simulink model "MMMS_v3"  (R2024b)
settings: Solver=VariableStepAuto  StartTime=0.0  StopTime=60  FixedStep=0.001  RelTol=1e-3
InitFcn:
  | %rho_0t=[0.29;0.29;0.29]; %m
  | %V_0t=[-0.001;-0.001;0];%[-0.0005;-0.0005;0];
  | %w_t=[0;0;-0.002];
  | 
  | 
  | %rho_0t=[0.3;0.3;0.2]; %m
  | %V_0t=[-0.001;-0.001;0];%[-0.0005;-0.0005;0];
  | %w_t=[0;0;-0.001];
values from neighbouring files (symbols this model uses):
  Dt = 0.1    [main_EKF.m]
  Fake_Manip_grad = -0.2.*eye(7)    [Initiate_FQ.m]
  g_cm = zeros(4,4,n)    [Initiate_KUKA_inv.m]    (also in Main_MMMS.m; test_KUKA_elements.m)
  g_It00 = [eye(3) rho_It;0 0 0 1]    [main_EKF.m]
  iota0 = eye(6,6)    [Initiate_KUKA_inv.m]    (also in Main_MMMS.m; test_KUKA_elements.m)
  K_d = 10*[1.3*eye(3) zeros(3);zeros(3) 0.8*eye(3)]    [Initiate_FQ.m]    (also in Initiate_KUKA_inv.m = 5*[0.7*eye(3) zeros(3);zeros(3) 0.5*eye(3)]; MMMS_Initiate_FQ.m; Main_MMMS.m = 5*[0.7*eye(3) zeros(3);zeros(3) 0.5*eye(3)]; test_KUKA_elements.m = 50*[0.7*eye(3) zeros(3);zeros(3) 0.5*eye(3)])
  K_i = 5*[0.1*eye(3) zeros(3);zeros(3) 0.01*eye(3)]    [Initiate_FQ.m]    (also in Initiate_KUKA_inv.m = 5*[0.01*eye(3) zeros(3);zeros(3) 0.001*eye(3)]; MMMS_Initiate_FQ.m; Main_MMMS.m = 5*[0.01*eye(3) zeros(3);zeros(3) 0.001*eye(3)]; test_KUKA_elements.m = 50*[0.01*eye(3) zeros(3);zeros(3) 0.001*eye(3)])
  K_p = 100*[0.1 0 0 0 0 0;0 0.1 0 0 0 0; 0 0 0.1 0 0 0; 0 0 0 0.01 0 0 ... (first row only)    [Initiate_FQ.m]    (also in Initiate_KUKA_inv.m = 5*[0.1 0 0 0 0 0;0 0.1 0 0 0 0; 0 0 0.1 0 0 0; 0 0 0 0.01 0 ; MMMS_Initiate_FQ.m; Main_MMMS.m = 5*[0.1 0 0 0 0 0;0 0.1 0 0 0 0; 0 0 0.1 0 0 0; 0 0 0 0.01 0 ; test_KUKA_elements.m = 50*[0.1 0 0 0 0 0;0 0.1 0 0 0 0; 0 0 0.1 0 0 0; 0 0 0 0.01 0)
  K_w = 200*eye(7)    [Initiate_FQ.m]    (also in MMMS_Initiate_FQ.m)
  K_wd = 2*eye(7)    [Initiate_FQ.m]    (also in MMMS_Initiate_FQ.m)
  m = randn(s,total_time_steps,6)*chol(R)    [main_EKF.m]
  M0 = M_temp.M0.data(:,:,1)    [Initiate_FQ.m]    (also in MMMS_Initiate_FQ.m; test_KUKA_elements.m)
  m0 = robot.Bodies{1,n+1}.Mass    [Initiate_KUKA_inv.m]    (also in Main_MMMS.m; test_KUKA_elements.m)
  m0_frak = diag_M(1:6,1:6)    [Initiate_KUKA_inv.m]    (also in Main_MMMS.m; make_uncertain.m = diag_M_unc(1:6,1:6); test_KUKA_elements.m)
  M0m = M_temp.M0m.data(:,:,1)    [Initiate_FQ.m]    (also in MMMS_Initiate_FQ.m; test_KUKA_elements.m)
  m_diag = diag_M(7:end,7:end)    [Initiate_KUKA_inv.m]    (also in Main_MMMS.m; make_uncertain.m = diag_M_unc(7:end,7:end); test_KUKA_elements.m)
  M_t = (((Adjoint(g_It))'\M_t_body)/(Adjoint(g_It)))    [Initiate_FQ.m]    (also in Initiate_KUKA_inv.m = [eye(3)*mt zeros(3); zeros(3) eye(3)*80]; MMMS_Initiate_FQ.m; Main_MMMS.m = [eye(3)*mt zeros(3); zeros(3) eye(3)*80]; test_KUKA_elements.m = [eye(3)*mt zeros(3); zeros(3) eye(3)*80])
  M_t_body = [eye(3)*mt zeros(3); zeros(3) eye(3)*0.416667]    [Initiate_FQ.m]    (also in MMMS_Initiate_FQ.m)
  mm = zeros(1,n)    [Initiate_KUKA_inv.m]    (also in Main_MMMS.m; test_KUKA_elements.m)
  mu = P0    [Initiate_FQ.m]    (also in Initiate_KUKA_inv.m = zeros(6,1); MMMS_Initiate_FQ.m; Main_MMMS.m = zeros(6,1); make_uncertain.m = P0_unc)
  mu_t = inv((Adjoint(g_It))')*M_t_body*[V_It;w_t]    [Initiate_FQ.m]    (also in Initiate_KUKA_inv.m = M_t*[V_0t;w_t]; MMMS_Initiate_FQ.m; Main_MMMS.m = M_t*[V_0t;w_t]; make_uncertain.m = inv((Adjoint(g_It))')*M_t_body_unc*[V_It;w_t])
  noise_st = 0.000005    (= 5e-06)    [main_EKF.m]
  q_dot_m = [0;0;0;0;0;0;0]    [Initiate_FQ.m]    (also in Initiate_KUKA_inv.m; MMMS_Initiate_FQ.m; Main_MMMS.m; test_KUKA_elements.m = [0])
  q_m = [0.2;1.2;0.3;2.5;0.5;1.5;0.6]    [Initiate_FQ.m]    (also in Initiate_KUKA_inv.m = [0;0;0;0;0;0;0]; MMMS_Initiate_FQ.m = [0.2;0.2;0.3;0.5;0.5;0.5;0.6]; Main_MMMS.m = [0;0;0;0;0;0;0]; test_KUKA_elements.m = [0.2;1.2;0.3;1.8;0.5;1.3;0.6])
  rho_It = [0;0;1.7]    [Initiate_FQ.m]    (also in MMMS_Initiate_FQ.m)
  s = RandStream.create('mrg32k3a','NumStreams',1)    [main_EKF.m]
  sc_size = 1    [Initiate_KUKA_inv.m]    (also in Main_MMMS.m; test_KUKA_elements.m)
  V_It = [0.0005;0.0005;0]    [Initiate_FQ.m]    (also in MMMS_Initiate_FQ.m = [0.001;0.001;0])
  Xi_m_matrix = zeros(6*n,n)    [Initiate_KUKA_inv.m]    (also in Main_MMMS.m)
undefined symbols (not defined in the file or in its folder): g_cm0, I0, Im, Mm, X, Xi_m, Y, Z
libraries: nesl_utility x314, sm_lib x231, robotcorelib x30, simulink x12
(part 13 of 13)

== matlab function MMMS_v3/Feedback Transformation2/Inverse Dynamics1/C_hat1/M_partials1/M0mpartial ==
  data: q_m input; M0m_partial output; V input; Lm input; Lm0 input; iota0 input; diag_Mm input; Lm0_partial input; Lm_partial input; Xi_m_matrix input
function M0m_partial = M0m_partial(q_m,V,Lm,Lm0,iota0,diag_Mm,Lm0_partial,Lm_partial, Xi_m_matrix)
% Calculates the C_hat_m matrix from base pose and arm joint angles

n=length(q_m);
b=length(V);

% Find partial of M0m to joint angles
M0m_partial=zeros(b,n,n);
for i=1:n
    temp1=transpose(Lm0_partial(1:end,1:end,i))*diag_Mm*Lm;
    temp2=transpose(Lm0)*diag_Mm*Lm_partial(1:end,1:end,i);
    M0m_partial(1:b,1:n,i)= iota0'*(temp1+temp2)*Xi_m_matrix; % equation 118 of TRO paper
end

== matlab function MMMS_v3/Feedback Transformation2/Inverse Dynamics1/C_hat1/M_partials1/M0mpartial_par ==
  data: q_m input; M0m_partial_par output; V input; Lm input; Lm0 input; iota0 input; diag_Mm input; Lm0_partial input; Lm_partial input; Xi_m_matrix input; Lm0_partial_par input; Lm_partial_par input
function M0m_partial_par = M0m_partial_par(q_m,V,Lm,Lm0,iota0,diag_Mm,Lm0_partial,Lm_partial, Xi_m_matrix,Lm0_partial_par,Lm_partial_par)
% Calculates the C_hat_m matrix from base pose and arm joint angles

n=length(q_m);
b=length(V);

% Find partial of M0m to joint angles
M0m_partial_par=zeros(b,n,n,n);
for i=1:n
    for s=1:n
        temp1=transpose(Lm0_partial_par(1:end,1:end,i,s))*diag_Mm*Lm;
        temp2=transpose(Lm0_partial(1:end,1:end,i))*diag_Mm*Lm_partial(1:end,1:end,s);
        temp3=transpose(Lm0_partial(1:end,1:end,s))*diag_Mm*Lm_partial(1:end,1:end,i);
        temp4=transpose(Lm0)*diag_Mm*Lm_partial_par(1:end,1:end,i,s);
        M0m_partial_par(1:b,1:n,i,s)= iota0'*(temp1+temp2+temp3+temp4)*Xi_m_matrix; % equation 118 of TRO paper
    end
end


% M0m_partial_par

== matlab function MMMS_v3/Feedback Transformation2/Inverse Dynamics1/C_hat1/M_partials1/Mmpartial ==
  data: q_m input; Mm_partial output; Xi_m_matrix input; Lm input; diag_Mm input; Lm_partial input
function Mm_partial = Mm_partial(q_m,Xi_m_matrix,Lm,diag_Mm,Lm_partial)
% Calculates the C_hat_m matrix from base pose and arm joint angles

n=length(q_m);

% find the non-generalized arm mass matrix'x derivative to joint angles
Mm_partial=zeros(n,n,n);
for i=1:n
    temp=   transpose(Lm_partial(1:6*n,1:6*n,i))*diag_Mm*Lm  +   transpose(Lm)*diag_Mm*Lm_partial(1:6*n,1:6*n,i);
    Mm_partial(1:n,1:n,i)=transpose(Xi_m_matrix)*temp*Xi_m_matrix; %calcualte the derivative of not-augmented arm mass matrix from equation 120 of TRO paper
end

== matlab function MMMS_v3/Feedback Transformation2/Inverse Dynamics1/C_hat1/Mm_hat_partial1 ==
  data: q_m input; AMA_partial input; Mm_hat_partial output; Mm_partial input
function Mm_hat_partial = Mm_hat_partial(q_m, AMA_partial, Mm_partial)
% Calculates the C_hat_m matrix from base pose and arm joint angles

n=length(q_m);

% find the generalized arm mass matrix'x derivative to joint angles
Mm_hat_partial=zeros(n,n,n);
for i=1:n
    Mm_hat_partial(1:n,1:n,i)=Mm_partial(1:n,1:n,i)-AMA_partial(1:n,1:n,i); %calcualte the derivative of augmented arm mass matrix from equation 119 of TRO paper
end

== matlab function MMMS_v3/Controller23/sensing noise in g_t ==
  data: err input; errM output
function errM = fcn(err)

errM=expm(wedge(err));

== matlab function MMMS_v3/Inverse Dynamics/N_hat1/MATLAB Function ==
  data: g_I0 input; V_Ie output; V_Ie_e input
function V_Ie = fcn(g_I0,V_Ie_e)

V_Ie = Adjoint(g_I0)\V_Ie_e;

== matlab function MMMS_v3/Controller23/V_It_2 ==
  data: mu_t input; M_t_body input; g_It input; V_It_2 output
function V_It_2 = V_It(mu_t, M_t_body, g_It)


% g_gpt=[eye(3) [0.25; 0.25; 0.25]; 0 0 0 1];
R=g_It(1:3,1:3);

% Pt=(Adjoint(g_It))'*mu_t;
V_It_2=(Adjoint(g_It))*inv(M_t_body)*(Adjoint(g_It)')*mu_t;%Adjoint(g_It)*M_t_body\Pt;%(Mt\(Adjoint(g_It)')*Pt); %[R zeros(3);zeros(3) R]



% Ad g_Igp(t) M^-1 Ad gI_gp(t)' inv(Ad g_I_gp') Mt inv (Ad g_I_gp) V_Igp

== matlab function MMMS_v3/Inverse Dynamics/C_hat1/AMA_partial ==
  data: q_m input; AMA_partial output; M0 input; A input; A_partial input; V input; M0_partial input
function AMA_partial = AMA_partial(q_m,M0,A,A_partial,V,M0_partial)
% Calculates the C_hat_m matrix from base pose and arm joint angles

n=length(q_m);
b=length(V);

% find the temp intermediate term
AMA_partial=zeros(n,n,n);
for i=1:n
    AMA_partial(1:n,1:n,i)=transpose(A_partial(1:end,1:end,i))*M0*A+transpose(A)*M0_partial(1:end,1:end,i)*A+transpose(A)*M0*A_partial(1:end,1:end,i); %calcualte the derivative of not-augmented arm mass matrix from equation 121 of TRO paper
end

== matlab function MMMS_v3/Inverse Dynamics/C_hat1/A_partial ==
  data: q_m input; A_partial output; M0 input; M0_partial input; M0m_partial input; M0m input; V input
function A_partial = A_partial(q_m,M0,M0_partial,M0m_partial,M0m,V)
% Calculates the C_hat_m matrix from base pose and arm joint angles

n=length(q_m);
b=length(V);

% Find partial of connection A to each joint angle
A_partial=zeros(b,n,n);

temp1=zeros(b,n);
temp2=zeros(b,n);
temp3=zeros(b,n);

for i=1:n
    temp1=M0\M0_partial(1:end,1:end,i);
    temp2=M0\M0m;
    temp3=M0\M0m_partial(1:end,1:end,i);
    A_partial(1:b,1:n,i)=-temp1*temp2+temp3; % Equation 122
end

== matlab function MMMS_v3/Controller23/Potential Function ==
  data: U_ff output; A input; w input; grad_w input; U_c input; p_0n input; sc_size input; Mm_hat input; g_n0 input
function U_ff = U_ff(A,w,grad_w, U_c, p_0n, sc_size,Mm_hat, g_n0)


grad_w_p=p_0n/(norm(p_0n)); % d/dt(1/sqrt(x^2+y^2+z^2)) = -1/2*w_p^3 * d/dt (x^2+...)
w_lim=0.003;
w_p_lim=0.02;
r_lim=sqrt(2)*sc_size/2+0.02;

w_p=norm(p_0n)-r_lim;

JJ=A;
A_dagger = ((Mm_hat)\JJ')/((JJ/Mm_hat)*JJ');

if w<w_lim %--------------------------------------------- close to singular
%     temp=(pinv(A)'*grad_w);
%     dir=(temp)./(norm(temp));
%     Uc=U_c-dot(U_c,dir).*dir;

    if w_p<w_p_lim %-------------- EE collision w Spacecraft
        if w_p<w_p_lim/4
            U_c=U_c-dot(U_c,[(grad_w_p); zeros(3,1)]);
        end
        U_c=U_c-10.*(1-w_p_lim/w_p)*((w_p_lim)/w_p^2).*[(grad_w_p); zeros(3,1)]; %(1/(1+100*exp(1000*(w_p-(sqrt(2)*sc_size/2+0.05)))))*2*
    end
    
    U_ff=U_c-((1-w_lim/w)*(w_lim/w^2).*A_dagger'*grad_w); %1*(1-w_lim/w)*
    %(1/(1+100*exp(1000*(w-0.003))))*0.0001*pinv(A)'*(-grad_w./(w^2)); 
    %adjoint_low(Adjoint(g_I0)*V_Ie)*Adjoint(inv(g_I0))*V_It+Adjoint(inv(g_I0))*V_It_dot

else %----------------------------------------------- NOT close to singular
    
    if w_p<w_p_lim %-------------- EE collision w Spacecraft
        if w_p<w_p_lim/4
            U_c=U_c-dot(U_c,[(grad_w_p); zeros(3,1)]);
        end
        U_c=U_c-10.*(1-w_p_lim/w_p)*((w_p_lim)/w_p^2).*[(grad_w_p); zeros(3,1)];
        %(1/(1+100*exp(1000*(w_p-(sqrt(2)*sc_size/2+0.05)))))*2*
        
    end

    U_ff=U_c;
end

== matlab function MMMS_v3/Controller23/mu_init ==
  data: g_It input; Mt input; V_It input; mu_init output
function mu_init = mu_init(g_It,Mt,V_It)

mu_init=Mt*V_It; %*(inv(Adjoint(g_It)))


% Ad g_Igp(t) M^-1 Ad gI_gp(t)' inv(Ad g_I_gp') Mt inv (Ad g_I_gp) V_Igp

== matlab function MMMS_v3/Controller23/V_It_1 ==
  data: V_It input; g_It input; V_It_3 output
function V_It_3 = V_It3(V_It, g_It)


% g_gpt=[eye(3) [0.25; 0.25; 0.25]; 0 0 0 1];
R=g_It(1:3,1:3);

V_It_3=Adjoint(g_It)*[R zeros(3);zeros(3) R]'*V_It; %[R zeros(3);zeros(3) R]


% Ad g_Igp(t) M^-1 Ad gI_gp(t)' inv(Ad g_I_gp') Mt inv (Ad g_I_gp) V_Igp

== matlab function MMMS_v3/Controller23/Kinematics/MATLAB Function ==
  data: g_I0 input; V_Ie output; V_Ie_e input
function V_Ie = fcn(g_I0,V_Ie_e)

V_Ie = Adjoint(g_I0)*V_Ie_e;

== matlab function MMMS_v3/Controller23/Filter/sensing noise in g_t1 ==
  data: z input; errM output; z_gt input
function errM = fcn(z,z_gt)

g_te=(z\z_gt);

R_te=g_te(1:3,1:3);
p_te=g_te(1:3,4);

temp_R=eye(3)-R_te;
temp_R=0.5*trace(temp_R);

temp_p=0.5*transpose(p_te)*p_te;
errM =temp_R+temp_p;

== matlab function MMMS_v3/Dynamic Parameters/ 1 ==
  data: q_m input; L0 output; Lm0 output; Lm output; Xi_m input
function [L0,Lm0,Lm] =L_calculator(q_m,Xi_m)
% Calculates the time-dependent L matrix
n=length(q_m);
L=zeros(6*(n+1),6*(n+1));
% Compute M_frak for ith body
% Calculate L matrix
for i=1:n+1
    for j=1:n+1
        if i>j
            Ad_temp=eye(6);
            for k=j:i-1
                Ad_temp=Adjoint(g_Matrix(-Xi_m(:,k),q_m(k)))*Ad_temp;
            end
            L(6*(i-1)+1:6*(i-1)+6,6*(j-1)+1:6*(j-1)+6)=Ad_temp;
        elseif i==j
            L(6*(i-1)+1:6*(i-1)+6,6*(j-1)+1:6*(j-1)+6)=eye(6);
        elseif i<j
            L(6*(i-1)+1:6*(i-1)+6,6*(j-1)+1:6*(j-1)+6)=zeros(6);
        end
    end
end

L0=L(1:6,1:6);
Lm0=L(7:end,1:6);
Lm=L(7:end,7:end);

end

== matlab function MMMS_v3/Controller23/Filter/sensing noise in g_t2 ==
  data: z input; errM output; z_gt input
function errM = fcn(z,z_gt)

g_te=(z\z_gt);

R_te=g_te(1:3,1:3);
p_te=g_te(1:3,4);

temp_R=eye(3)-R_te;
temp_R=0.5*trace(temp_R);

temp_p=0.5*transpose(p_te)*p_te;
errM =temp_R+temp_p;

== matlab function MMMS_v3/Inverse Dynamics/C_hat1/C_hat ==
  data: q_m input; Mm_hat_partial input; q_dot_m input; C_hat output
function C_hat = C_hat(q_m, Mm_hat_partial,q_dot_m)
% Calculates the C_hat_m matrix from base pose and arm joint angles

n=length(q_m);


% Calculate C_hat matrix
C_temp1=zeros(n,n);
C_temp2=zeros(n,n);
C_hat=zeros(n,n);
for i=1:n
    C_temp1=C_temp1+squeeze(Mm_hat_partial(1:n,1:n,i)).*q_dot_m(i); % nxn by scalar
    C_temp2(i,1:n)=0.5*transpose(q_dot_m)*squeeze(Mm_hat_partial(1:n,1:n,i)); %1xn by nxn 
end

C_hat=C_temp1-C_temp2;

== matlab function MMMS_v3/Controller23/  ==
  data: A input; normA output
function normA  = normA(A)

normA=norm(A);

== matlab function MMMS_v3/MMS3/collect positions ==
  data: p_ni output; p_n2 input; p_n3 input; p_n4 input; p_n5 input; g_n0 input
function p_ni = collect_positions(p_n2,p_n3,p_n4,p_n5, g_n0)

% R_0n=g_n0(1:3,1:3);
% p_0n=g_n0(1:3,4);

% p_joints=zeros(3,5);
p_ni=[p_n2 p_n3 p_n4  p_n5];
% p_joints=p_joints_temp(1:3,:);

== matlab function MMMS_v3/MMS3/collect positions1 ==
  data: g_ni output; g_n2 input; g_n3 input; g_n4 input; g_n5 input; g_n0 input
function g_ni = collect_poses(g_n2,g_n3,g_n4,g_n5, g_n0)

g_ni=zeros(4,4,4);
% p_joints=zeros(3,5);
g_ni(1,:,:)=g_n2;
g_ni(2,:,:)=g_n3;
g_ni(3,:,:)=g_n4;
g_ni(4,:,:)=g_n5;

== matlab function MMMS_v3/MMS4/collect positions ==
  data: p_ni output; p_n2 input; p_n3 input; p_n4 input; p_n5 input; g_n0 input
function p_ni = collect_positions(p_n2,p_n3,p_n4,p_n5, g_n0)

% R_0n=g_n0(1:3,1:3);
% p_0n=g_n0(1:3,4);

% p_joints=zeros(3,5);
p_ni=[p_n2 p_n3 p_n4  p_n5];
% p_joints=p_joints_temp(1:3,:);

== matlab function MMMS_v3/Inverse Dynamics/C_hat1/Lm_partials/Lm0partial ==
  data: q_m input; Lm0_partial output; Xi_m input; iota0 input
function Lm0_partial = Lm0_partial(q_m,Xi_m,iota0)
% Calculates the C_hat_m matrix from base pose and arm joint angles

n=length(q_m);

% Find partial of Lm to joint angles
Lm0_partial=zeros(6*n,6,n); % 6nx6xn
for i=1:n
    for j=1:n
        Lm0_partial(6*(j-1)+1:6*j,1:6,i)=Ad_partial(j,1,i,Xi_m,q_m,iota0); % equation 114 of TRO paper
    end
end

%%%%%%%%%%%%%%%%%%%%%%%%%%%%%%%%%%%%%%%%%%%%%%%%%%%%%%%%%%%%% MUST BE
%%%%%%%%%%%%%%%%%%%%%%%%%%%%%%%%%%%%%%%%%%%%%%%%%%%%%%%%%%%%% CHECKED

== matlab function MMMS_v3/MMS4/collect positions1 ==
  data: g_ni output; g_n2 input; g_n3 input; g_n4 input; g_n5 input; g_n0 input
function g_ni = collect_poses(g_n2,g_n3,g_n4,g_n5, g_n0)

g_ni=zeros(4,4,4);
% p_joints=zeros(3,5);
g_ni(1,:,:)=g_n2;
g_ni(2,:,:)=g_n3;
g_ni(3,:,:)=g_n4;
g_ni(4,:,:)=g_n5;

== matlab function MMMS_v3/Controller1/  ==
  data: A input; normA output
function normA  = normA(A)

normA=norm(A);

== matlab function MMMS_v3/Dynamic Parameters1/ 1 ==
  data: q_m input; L0 output; Lm0 output; Lm output; Xi_m input
function [L0,Lm0,Lm] =L_calculator(q_m,Xi_m)
% Calculates the time-dependent L matrix
n=length(q_m);
L=zeros(6*(n+1),6*(n+1));
% Compute M_frak for ith body
% Calculate L matrix
for i=1:n+1
    for j=1:n+1
        if i>j
            Ad_temp=eye(6);
            for k=j:i-1
                Ad_temp=Adjoint(g_Matrix(-Xi_m(:,k),q_m(k)))*Ad_temp;
            end
            L(6*(i-1)+1:6*(i-1)+6,6*(j-1)+1:6*(j-1)+6)=Ad_temp;
        elseif i==j
            L(6*(i-1)+1:6*(i-1)+6,6*(j-1)+1:6*(j-1)+6)=eye(6);
        elseif i<j
            L(6*(i-1)+1:6*(i-1)+6,6*(j-1)+1:6*(j-1)+6)=zeros(6);
        end
    end
end

L0=L(1:6,1:6);
Lm0=L(7:end,1:6);
Lm=L(7:end,7:end);

end

== matlab function MMMS_v3/Dynamic Parameters1/MATLAB Function ==
  data: A input; wt output
function wt = fcn(A)

J=-A;
% SVD=svd(J);

% minSVD=min(SVD);
% maxSVD=max(SVD);

wt=sqrt(det(J*J'));

% y = minSVD/maxSVD;

== matlab function MMMS_v3/Controller23/gradient_of_Eg ==
  data: g_te input; Nabla_Eg output
function Nabla_Eg = fcn(g_te)

% Calculate the gradient of the Pose Error Function
p_te=g_te(1:3,4);
R_te=g_te(1:3,1:3);

temp=0.5*(R_te-transpose(R_te));

R_temp=vee3(temp);

Nabla_Eg=[p_te;R_temp];

== matlab function MMMS_v3/Inverse Dynamics/C_hat1/Lm_partials/Lmpartial ==
  data: q_m input; Lm_partial output; Xi_m input; iota0 input
function Lm_partial  = Lm_partial(q_m,Xi_m,iota0)
% Calculates the C_hat_m matrix from base pose and arm joint angles

n=length(q_m);

% Find partial of Lm0 to joint angles
Lm_partial=zeros(6*n,6*n,n); % 6nx6xn
for i=1:n
    Lm_partial(:,:,i)=zeros(6*n,6*n);
    for j=2:n
        for k=2:n
            if j>i && i>=k
                Lm_partial(6*(j-1)+1:6*j,6*(k-2)+1:6*(k-1),i)=Ad_partial(j,k,i,Xi_m,q_m,iota0); % equation 81 of TRO paper
            elseif i==j && i>=k
                Lm_partial(6*(j-1)+1:6*j,6*(k-2)+1:6*(k-1),i)=Ad_partial(j,k,i,Xi_m,q_m,iota0); % equation 81 of TRO paper
            else
                Lm_partial(6*(j-1)+1:6*(j-1)+6,6*(k-2)+1:6*(k-2)+6,i)=zeros(6,6);
            end

        end
    end
end

== matlab function MMMS_v3/Inverse Dynamics/C_hat1/M_partials/ M0partial ==
  data: q_m input; M0_partial output; Lm0 input; V input; iota0 input; diag_Mm input; Lm0_partial input
function M0_partial = M0_partial(q_m,Lm0,V,iota0,diag_Mm,Lm0_partial)
% Calculates the C_hat_m matrix from base pose and arm joint angles

n=length(q_m);
b=length(V);

% Find partial of M0 to joint angles
M0_partial=zeros(b,b,n); %initiate
for i=1:n
    temp1=transpose(Lm0_partial(1:end,1:end,i))*diag_Mm*Lm0;
    temp2=transpose(Lm0)*diag_Mm*Lm0_partial(1:end,1:end,i);
    M0_partial(1:b,1:b,i)= iota0'*(temp1+temp2)*iota0; %6x6 %equation 117 of TRO
end

== matlab function MMMS_v3/Inverse Dynamics/C_hat1/M_partials/M0mpartial ==
  data: q_m input; M0m_partial output; V input; Lm input; Lm0 input; iota0 input; diag_Mm input; Lm0_partial input; Lm_partial input; Xi_m_matrix input
function M0m_partial = M0m_partial(q_m,V,Lm,Lm0,iota0,diag_Mm,Lm0_partial,Lm_partial, Xi_m_matrix)
% Calculates the C_hat_m matrix from base pose and arm joint angles

n=length(q_m);
b=length(V);

% Find partial of M0m to joint angles
M0m_partial=zeros(b,n,n);
for i=1:n
    temp1=transpose(Lm0_partial(1:end,1:end,i))*diag_Mm*Lm;
    temp2=transpose(Lm0)*diag_Mm*Lm_partial(1:end,1:end,i);
    M0m_partial(1:b,1:n,i)= iota0'*(temp1+temp2)*Xi_m_matrix; % equation 118 of TRO paper
end

== matlab function MMMS_v3/Inverse Dynamics/C_hat1/M_partials/Mmpartial ==
  data: q_m input; Mm_partial output; Xi_m_matrix input; Lm input; diag_Mm input; Lm_partial input
function Mm_partial = Mm_partial(q_m,Xi_m_matrix,Lm,diag_Mm,Lm_partial)
% Calculates the C_hat_m matrix from base pose and arm joint angles

n=length(q_m);

% find the non-generalized arm mass matrix'x derivative to joint angles
Mm_partial=zeros(n,n,n);
for i=1:n
    temp=   transpose(Lm_partial(1:6*n,1:6*n,i))*diag_Mm*Lm  +   transpose(Lm)*diag_Mm*Lm_partial(1:6*n,1:6*n,i);
    Mm_partial(1:n,1:n,i)=transpose(Xi_m_matrix)*temp*Xi_m_matrix; %calcualte the derivative of not-augmented arm mass matrix from equation 120 of TRO paper
end

== matlab function MMMS_v3/Inverse Dynamics/C_hat1/Mm_hat_partial ==
  data: q_m input; AMA_partial input; Mm_hat_partial output; Mm_partial input
function Mm_hat_partial = Mm_hat_partial(q_m, AMA_partial, Mm_partial)
% Calculates the C_hat_m matrix from base pose and arm joint angles

n=length(q_m);

% find the generalized arm mass matrix'x derivative to joint angles
Mm_hat_partial=zeros(n,n,n);
for i=1:n
    Mm_hat_partial(1:n,1:n,i)=Mm_partial(1:n,1:n,i)-AMA_partial(1:n,1:n,i); %calcualte the derivative of augmented arm mass matrix from equation 119 of TRO paper
end

== matlab function MMMS_v3/Dynamic Parameters1/MATLAB Function1 ==
  data: g_I0 input; mu input; P output
function P=Momentum(g_I0,mu)
% find the momentum in current base frame
P=Adjoint(g_I0)'*mu;

== matlab function MMMS_v3/Controller23/Kinematics/V_It_1 ==
  data: V_I0 input; g_I0 input; V_I0_3 output
function V_I0_3 = V_I03(V_I0, g_I0)


% g_gpt=[eye(3) [0.25; 0.25; 0.25]; 0 0 0 1];
R=g_I0(1:3,1:3);

V_I0_3=Adjoint(g_I0)*[R zeros(3);zeros(3) R]'*V_I0; %[R zeros(3);zeros(3) R]


% Ad g_Igp(t) M^-1 Ad gI_gp(t)' inv(Ad g_I_gp') Mt inv (Ad g_I_gp) V_Igp

== matlab function MMMS_v3/Controller1/Kinematics/MATLAB Function ==
  data: g_I0 input; V_Ie output; V_Ie_e input
function V_Ie = fcn(g_I0,V_Ie_e)

V_Ie = Adjoint(g_I0)*V_Ie_e;

== matlab function MMMS_v3/Controller13/Kinematics/Pose Error Function ==
  data: g_te input; E_g output
function E_g = pose_Error_function(g_te)
% Calculates the pose Error function from the relative pose of end-effector to target
R_te=g_te(1:3,1:3);
p_te=g_te(1:3,4);

temp_R=eye(3)-R_te;
temp_R=0*0.5*trace(temp_R); %% CHANGED

temp_p=0.5*transpose(p_te)*p_te;
E_g =temp_R+temp_p;

== matlab function MMMS_v3/Controller1/Kinematics/Pose Error Function ==
  data: g_te input; E_g output
function E_g = pose_Error_function(g_te)
% Calculates the pose Error function from the relative pose of end-effector to target
R_te=g_te(1:3,1:3);
p_te=g_te(1:3,4);

temp_R=eye(3)-R_te;
temp_R=0.5*trace(temp_R);

temp_p=0.5*transpose(p_te)*p_te;
E_g =temp_R+temp_p;

== matlab function MMMS_v3/Controller13/Kinematics/Velocity_error ==
  data: g_I0 input; V_Ie input; V_e output; V_It input; g_It input; normV output
function [V_e,normV] = Velocity_Error_function(g_I0, V_Ie,V_It, g_It)
% Calculates the Velocity Error function from the momentums of chaser and
% target and the joint velocities

Rt=g_It(1:3,1:3);
R0=g_I0(1:3,1:3);

V_te_I=V_Ie-V_It; %Adjoint(inv(g_I0))*
V_te=Adjoint(inv(g_I0))*V_te_I;
V_e=V_te;

normV=norm(V_e);

== matlab function MMMS_v3/Controller1/Kinematics/V_It_1 ==
  data: V_I0 input; g_I0 input; V_I0_3 output
function V_I0_3 = V_I03(V_I0, g_I0)


% g_gpt=[eye(3) [0.25; 0.25; 0.25]; 0 0 0 1];
R=g_I0(1:3,1:3);

V_I0_3=Adjoint(g_I0)*[R zeros(3);zeros(3) R]'*V_I0; %[R zeros(3);zeros(3) R]


% Ad g_Igp(t) M^-1 Ad gI_gp(t)' inv(Ad g_I_gp') Mt inv (Ad g_I_gp) V_Igp

== matlab function MMMS_v3/Controller1/Kinematics/Velocity_error ==
  data: g_I0 input; V_Ie input; V_e output; V_It input; g_It input; normV output
function [V_e,normV] = Velocity_Error_function(g_I0, V_Ie,V_It, g_It)
% Calculates the Velocity Error function from the momentums of chaser and
% target and the joint velocities

Rt=g_It(1:3,1:3);
R0=g_I0(1:3,1:3);

V_te_I=V_Ie-V_It; %Adjoint(inv(g_I0))*
V_te=Adjoint(inv(g_I0))*V_te_I;
V_e=V_te;

normV=norm(V_e);

== matlab function MMMS_v3/Controller1/Nullspace derivatives ==
  data: Mm input; A input; N_dot output; Mm_partial input; A_partial input; q_dot input; Z_dot output; j input; Nj input
function [N_dot,Z_dot] =Nullspace_derivatives(Mm,A,Mm_partial,A_partial,q_dot,j, Nj)

Mm_dot=zeros(7);
A_dot=zeros(6,7);
for i=1:length(Mm_partial(1,1,:))
    Mm_dot=Mm_dot+Mm_partial(:,:,i).*q_dot(i);
    A_dot=A_dot+A_partial(:,:,i).*q_dot(i);
end

%parts of N_dot

N1=((Mm\Mm_dot)/Mm)     *   A'   / ((A/Mm)*A')*A;
N2=-Mm\A_dot'   /   ((A/Mm)*A')   * A;
N3=(Mm\A')   /   ((A/Mm)*A')    * ((A_dot/Mm)*A'  -   (A/Mm) *(Mm_dot /Mm) *A'    +   (A/Mm)*A_dot') /   ((A/Mm)*A')   *   A;
N4=-(Mm\ A') *    ((A/Mm)*A')  *A_dot;

N_dot=N1+N2+N3+N4;

% Z_dot=N_dot(:,j);%/norm_Z;
Nj_dot=N_dot(:,j);

Z_dot=Nj_dot/norm(Nj)-Nj'*Nj_dot*Nj/norm(Nj)^3;

== matlab function MMMS_v3/Controller1/Nullspace_maps ==
  data: Mm input; A input; N output; q_dot_m input
function N  =Nullspace_maps(Mm,A,q_dot_m)

n=length(q_dot_m);

N_Am=eye(n)-(Mm\A') *   (   (   (A/Mm) *   A')\    A);
N=N_Am;

== matlab function MMMS_v3/Controller1/Potential Function ==
  data: U_ff output; A input; w input; grad_w input; U_c input; p_0n input; sc_size input; Mm_hat input; g_n0 input
function U_ff = U_ff(A,w,grad_w, U_c, p_0n, sc_size,Mm_hat, g_n0)


grad_w_p=p_0n/(norm(p_0n)); % d/dt(1/sqrt(x^2+y^2+z^2)) = -1/2*w_p^3 * d/dt (x^2+...)
w_lim=0.003;
w_p_lim=0.02;
r_lim=sqrt(2)*sc_size/2+0.02;

w_p=norm(p_0n)-r_lim;

JJ=A;
A_dagger = ((Mm_hat)\JJ')/((JJ/Mm_hat)*JJ');

if w<w_lim %--------------------------------------------- close to singular
%     temp=(pinv(A)'*grad_w);
%     dir=(temp)./(norm(temp));
%     Uc=U_c-dot(U_c,dir).*dir;

    if w_p<w_p_lim %-------------- EE collision w Spacecraft
        if w_p<w_p_lim/4
            U_c=U_c-dot(U_c,[(grad_w_p); zeros(3,1)]);
        end
        U_c=U_c;%-10.*(1-w_p_lim/w_p)*((w_p_lim)/w_p^2).*[(grad_w_p); zeros(3,1)]; %(1/(1+100*exp(1000*(w_p-(sqrt(2)*sc_size/2+0.05)))))*2*
    end
    
    U_ff=U_c-((1-w_lim/w)*(w_lim/w^2).*A_dagger'*grad_w); %1*(1-w_lim/w)*
    %(1/(1+100*exp(1000*(w-0.003))))*0.0001*pinv(A)'*(-grad_w./(w^2)); 
    %adjoint_low(Adjoint(g_I0)*V_Ie)*Adjoint(inv(g_I0))*V_It+Adjoint(inv(g_I0))*V_It_dot

else %----------------------------------------------- NOT close to singular
    
    if w_p<w_p_lim %-------------- EE collision w Spacecraft
        if w_p<w_p_lim/4
            U_c=U_c-dot(U_c,[(grad_w_p); zeros(3,1)]);
        end
        U_c=U_c;%-10.*(1-w_p_lim/w_p)*((w_p_lim)/w_p^2).*[(grad_w_p); zeros(3,1)];
        %(1/(1+100*exp(1000*(w_p-(sqrt(2)*sc_size/2+0.05)))))*2*
        
    end

    U_ff=U_c;
end

== matlab function MMMS_v3/Dynamic Parameters/MATLAB Function ==
  data: A input; wt output
function wt = fcn(A)

J=-A;
% SVD=svd(J);

% minSVD=min(SVD);
% maxSVD=max(SVD);

wt=sqrt(det(J*J'));

% y = minSVD/maxSVD;

== matlab function MMMS_v3/Controller13/V_It_1 ==
  data: V_It input; g_It input; V_It_3 output
function V_It_3 = V_It3(V_It, g_It)


% g_gpt=[eye(3) [0.25; 0.25; 0.25]; 0 0 0 1];
R=g_It(1:3,1:3);

V_It_3=Adjoint(g_It)*[R zeros(3);zeros(3) R]'*V_It; %[R zeros(3);zeros(3) R]


% Ad g_Igp(t) M^-1 Ad gI_gp(t)' inv(Ad g_I_gp') Mt inv (Ad g_I_gp) V_Igp

== matlab function MMMS_v3/Controller13/V_It_2 ==
  data: mu_t input; M_t_body input; g_It input; V_It_2 output
function V_It_2 = V_It(mu_t, M_t_body, g_It)


% g_gpt=[eye(3) [0.25; 0.25; 0.25]; 0 0 0 1];
R=g_It(1:3,1:3);

% Pt=(Adjoint(g_It))'*mu_t;
V_It_2=(Adjoint(g_It))*inv(M_t_body)*(Adjoint(g_It)')*mu_t;%Adjoint(g_It)*M_t_body\Pt;%(Mt\(Adjoint(g_It)')*Pt); %[R zeros(3);zeros(3) R]



% Ad g_Igp(t) M^-1 Ad gI_gp(t)' inv(Ad g_I_gp') Mt inv (Ad g_I_gp) V_Igp

== matlab function MMMS_v3/Controller13/Velocity_error1 ==
  data: w input; out output; in input
function out = cut_off(w, in)

if w<0.003
    out=0.*in; %adjoint_low(Adjoint(g_I0)*V_Ie)*Adjoint(inv(g_I0))*V_It+Adjoint(inv(g_I0))*V_It_dot
else
    out=in;
end

== matlab function MMMS_v3/Controller1/Potential Function1 ==
  data: w_p output; p_0n input
function w_p = norm( p_0n)

w_p=norm(p_0n);

== matlab function MMMS_v3/Controller1/Potential Function3 ==
  data: f_pot output; p_ni input; g_ni input; sc_size input; g_n0 input; A input; p_i output
function [f_pot,p_i]  = potential_joints( p_ni, g_ni, sc_size, g_n0, A)

% w_joints=zeros(1,4);
grad_p_joints=zeros(3,4);
grad_p=zeros(7,4);
f_pot=zeros(7,1);
gain=0.01.*[1 1 1 1];%*[70 70 70 70];

p_lim=0.05;
r_lim=sqrt(2)*sc_size/2;


p_i=[0;0;0;0];

for i=1:4
    p_i(i)=norm(p_ni(:,i))-r_lim; %X_e
end

J_joints=zeros(4,7,6);
tempj=zeros(4,4);
for i=1:4
    % J_joints(i,:,:)=Adjoint(inv(g_n0))*[A(:,1:i+1) 0.*A(:,i+2:end)];
    tempj(:,:)=g_ni(i,:,:);
    J_joints(i,:,:)=[0.*A(:,1:i+1) -A(:,i+2:end)]'*Adjoint(inv(g_n0\tempj))';
end

R=zeros(3,3);
temp=zeros(7,6);
norm_grad_p=zeros(4,1);
% temp2=zeros(4);
    for i=1:4 %------------------------------ Joints collision w Spacecraft
        % w_joints(i)=norm(p_joints(:,i));%+[0; 0; 0.15]);
        if p_i(i)>p_lim %|| p_i<0.001
            grad_p_joints(:,i)=zeros(3,1);
        elseif p_i(i)<=0 && p_i(i)>-p_lim
            grad_p_joints(:,i)=-(p_ni(:,i))/norm(p_ni(i));
        elseif p_i(i)<-p_lim
            grad_p_joints(:,i)=zeros(3,1);
        else
            grad_p_joints(:,i)=(p_ni(:,i))/norm(p_ni(i));
        end
        temp(:,:)=J_joints(i,:,:);
        
        % temp2=squeeze(g_ni(i,:,:));
        % temp3=g_n0*temp2;

        R(:,:)=g_ni(i,1:3,1:3);
        grad_p(:,i)=temp*[R'*grad_p_joints(:,i);zeros(3,1)];
        norm_grad_p(i)=norm(grad_p(:,i));
        
    
        if p_i(i)<p_lim
            f_pot=f_pot-gain(i)*(1-p_lim/p_i(i))*((p_lim)/(p_i(i))^2).*(grad_p(:,i));  %((1/(1+100*exp(1000*(-(sqrt(2)*sc_size/2+0.0)))))
        end
        
    end

== matlab function MMMS_v3/Inverse Dynamics/N_hat1/N_hat ==
  data: N_hat_temp output; q_m input; q_dot_m input; A input; V input; P input; M0_partial input; A_partial input; iota0 input; M0 input
function N_hat_temp = N_hat(q_m,q_dot_m,A,V,P,M0_partial, A_partial, iota0, M0)
% Calculates the N_hat_m matrix from base pose and arm joint angles

n=length(q_m);
b=length(V);

%Form N_hat from equation 19 of ACC paper
N_temp1=zeros(n,b); N_temp2=zeros(n,b); N_temp3=zeros(n,b);

for i=1:n
    N_temp1=N_temp1+transpose(squeeze(A_partial(1:b,1:n,i)).*q_dot_m(i)); % transpose of (bxn times 1x1) 
    N_temp2(i,1:b)=transpose(q_dot_m)*transpose(squeeze(A_partial(1:b,1:n,i))); %1xn times nxb
    N_temp3(i,1:b)=0.5*transpose(P)*(M0\squeeze(M0_partial(1:end,1:end,i)))/(M0); % 1xb times bxb
end

N_hat_temp=-transpose(A)*transpose(adjoint_low(V,iota0))-N_temp1+N_temp2+N_temp3;

== matlab function MMMS_v3/Controller1/V_It_1 ==
  data: V_It input; g_It input; V_It_3 output
function V_It_3 = V_It3(V_It, g_It)


% g_gpt=[eye(3) [0.25; 0.25; 0.25]; 0 0 0 1];
R=g_It(1:3,1:3);

V_It_3=Adjoint(g_It)*[R zeros(3);zeros(3) R]'*V_It; %[R zeros(3);zeros(3) R]


% Ad g_Igp(t) M^-1 Ad gI_gp(t)' inv(Ad g_I_gp') Mt inv (Ad g_I_gp) V_Igp

== matlab function MMMS_v3/Controller23/Kinematics/Pose Error Function ==
  data: g_te input; E_g output
function E_g = pose_Error_function(g_te)
% Calculates the pose Error function from the relative pose of end-effector to target
R_te=g_te(1:3,1:3);
p_te=g_te(1:3,4);

temp_R=eye(3)-R_te;
temp_R=0.5*trace(temp_R);

temp_p=0.5*transpose(p_te)*p_te;
E_g =temp_R+temp_p;

== matlab function MMMS_v3/Controller1/V_It_2 ==
  data: mu_t input; M_t_body input; g_It input; V_It_2 output
function V_It_2 = V_It(mu_t, M_t_body, g_It)


% g_gpt=[eye(3) [0.25; 0.25; 0.25]; 0 0 0 1];
R=g_It(1:3,1:3);

% Pt=(Adjoint(g_It))'*mu_t;
V_It_2=(Adjoint(g_It))*inv(M_t_body)*(Adjoint(g_It)')*mu_t;%Adjoint(g_It)*M_t_body\Pt;%(Mt\(Adjoint(g_It)')*Pt); %[R zeros(3);zeros(3) R]



% Ad g_Igp(t) M^-1 Ad gI_gp(t)' inv(Ad g_I_gp') Mt inv (Ad g_I_gp) V_Igp

== matlab function MMMS_v3/Controller13/gradient_of_Eg ==
  data: g_te input; Nabla_Eg output
function Nabla_Eg = fcn(g_te)

% Calculate the gradient of the Pose Error Function
p_te=g_te(1:3,4);
R_te=g_te(1:3,1:3);

temp=0.5*(R_te-transpose(R_te));

R_temp=vee3(temp);

Nabla_Eg=[p_te;R_temp];

== matlab function MMMS_v3/Controller1/Velocity_error1 ==
  data: w input; out output; in input
function out = cut_off(w, in)

if w<0.003
    out=0.*in; %adjoint_low(Adjoint(g_I0)*V_Ie)*Adjoint(inv(g_I0))*V_It+Adjoint(inv(g_I0))*V_It_dot
else
    out=in;
end

== matlab function MMMS_v3/Controller13/mu_init ==
  data: g_It input; Mt input; V_It input; mu_init output
function mu_init = mu_init(g_It,Mt,V_It)

mu_init=Mt*V_It; %*(inv(Adjoint(g_It)))


% Ad g_Igp(t) M^-1 Ad gI_gp(t)' inv(Ad g_I_gp') Mt inv (Ad g_I_gp) V_Igp

== matlab function MMMS_v3/Controller1/Z ==
  data: N input; Z output; Z_dagger output; Mm input; j output; Nj output
function [Z,Z_dagger,j,Nj] =Z(N,Mm)

% m=length(temp(1,:));
% 
% for i=1:m
%     Z(:,i)=Mm*temp(:,i);
% end
nN=zeros(7,1);
for j=1:7
    nN(j,1)=N(:,j)'*N(:,j);
end

[nmax,j]=max(nN);

Z=N(:,j)/norm(N(:,j));

Z_dagger=(Z'*Mm*Z)\(Z'*Mm);

norm_Z=norm(N(:,j));

Nj=N(:,j);

== matlab function MMMS_v3/Controller1/Z dagger derivative ==
  data: Z_dagger input; N_dot input; Z_dot_dagger output; Z_dot input
function Z_dot_dagger =Z_dot_dagger(Z_dagger,N_dot,Z_dot)

Z_dot_dagger=Z_dagger*N_dot-Z_dagger*Z_dot*Z_dagger;

== matlab function MMMS_v3/Controller1/ZKw ==
  data: Z input; K_w_grad_w input; out output
function out  =for_i(Z, K_w_grad_w)


out=Z'*K_w_grad_w;

== matlab function MMMS_v3/Controller1/grad w ==
  data: A input; grad_w output; A_partial input; q_dot input
function grad_w  = grad_w(A,A_partial, q_dot)

w=sqrt(det(A*A'));

n=length(q_dot);
grad_w=zeros(n,1);
for i=1:n
    grad_w(i) = w/2* trace(   (A*A')\(A*A_partial(:,:,i)'+A_partial(:,:,i)*A')    );%det(A*A')*trace(inv(A')A_dot'+inv(A')*inv(A)*A_dot*A');
end

% w_dot=1/norm(grad_w'*q_dot);

== matlab function MMMS_v3/Controller23/Kinematics/Velocity_error ==
  data: g_I0 input; V_Ie input; V_e output; V_It input; g_It input; normV output
function [V_e,normV] = Velocity_Error_function(g_I0, V_Ie,V_It, g_It)
% Calculates the Velocity Error function from the momentums of chaser and
% target and the joint velocities

Rt=g_It(1:3,1:3);
R0=g_I0(1:3,1:3);

V_te_I=V_Ie-V_It; %Adjoint(inv(g_I0))*
V_te=Adjoint(inv(g_I0))*V_te_I;
V_e=V_te;

normV=norm(V_e);

== matlab function MMMS_v3/Controller1/gradient_of_Eg ==
  data: g_te input; Nabla_Eg output
function Nabla_Eg = fcn(g_te)

% Calculate the gradient of the Pose Error Function
p_te=g_te(1:3,4);
R_te=g_te(1:3,1:3);

temp=0.5*(R_te-transpose(R_te));

R_temp=vee3(temp);

Nabla_Eg=[p_te;R_temp];

== matlab function MMMS_v3/Controller1/joint distance from spacecraft ==
  data: pnorm output; p_joints input
function pnorm = norm( p_joints)

pnorm=zeros(4,1);
for i=1:4
    pnorm(i)=norm(p_joints(:,i));
end

== matlab function MMMS_v3/Controller1/mu_init ==
  data: g_It input; Mt input; V_It input; mu_init output
function mu_init = mu_init(g_It,Mt,V_It)

mu_init=Mt*V_It; %*(inv(Adjoint(g_It)))


% Ad g_Igp(t) M^-1 Ad gI_gp(t)' inv(Ad g_I_gp') Mt inv (Ad g_I_gp) V_Igp

== matlab function MMMS_v3/Controller1/nullspace_mapping ==
  data: Mm input; K_w_grad_w input; q_dot_m input; Z input; Z_dagger input; f_N output; Z_dot_dagger input; K_nu_nu input; f_pot input; out2 output; fw_i input
function [f_N, out2] =null_space(Mm, K_w_grad_w, q_dot_m,Z, Z_dagger,Z_dot_dagger, K_nu_nu, f_pot, fw_i)

f_N=zeros(7,1);

% nu=Z_dagger*q_dot_m;


f_N=Mm*Z*(-Z_dot_dagger*q_dot_m-K_nu_nu+(1)*Z'*K_w_grad_w-0.*fw_i +1.*Z_dagger*f_pot);

out2=Z_dagger*K_w_grad_w;

% 
% for i=1:m
%     fw =fw+ dot(w_opt, null_space(:,i)) / norm(null_space(:,i))^2 * null_space(:,i);
% end

% for i=1:m
%     fw =fw+ dot(f_pot, null_space(:,i)) / norm(null_space(:,i))^2 * null_space(:,i);
% end

% A_dot=A_partial*q_dot;


% JJ=A/Mm;
% null_space=eye(7)-(JJ'/(JJ*JJ'))*JJ;
% fw=zeros(7,1);
% fw=fw+null_space*f_pot;
% f_N=fw+null_space*w_opt;

== matlab function MMMS_v3/Dynamic Parameters1/V_I1 ==
  data: P input; A_connection input; q_dot_m input; M0 input; V_I0 output; g_I0 input
function V_I0 = V_I0(P, A_connection, q_dot_m, M0, g_I0)
V_I0=Adjoint(g_I0)*((M0\P)-A_connection*q_dot_m);

== matlab function MMMS_v3/Feedback Transformation/Inverse Dynamics1/A_dot ==
  data: A_partial input; q_m_dot input; A_dot output
function A_dot = fcn(A_partial, q_m_dot)
n=length(q_m_dot);

A_dot=zeros(6,n);
for i=1:n
    A_dot=A_dot+A_partial(:,:,i).*q_m_dot(i);
end

== matlab function MMMS_v3/Feedback Transformation/Inverse Dynamics1/C_hat/AMA_partial ==
  data: q_m input; AMA_partial output; M0 input; A input; A_partial input; V input; M0_partial input
function AMA_partial = AMA_partial(q_m,M0,A,A_partial,V,M0_partial)
% Calculates the C_hat_m matrix from base pose and arm joint angles

n=length(q_m);
b=length(V);

% find the temp intermediate term
AMA_partial=zeros(n,n,n);
for i=1:n
    AMA_partial(1:n,1:n,i)=transpose(A_partial(1:end,1:end,i))*M0*A+transpose(A)*M0_partial(1:end,1:end,i)*A+transpose(A)*M0*A_partial(1:end,1:end,i); %calcualte the derivative of not-augmented arm mass matrix from equation 121 of TRO paper
end

== matlab function MMMS_v3/Feedback Transformation/Inverse Dynamics1/C_hat/A_partial ==
  data: q_m input; A_partial output; M0 input; M0_partial input; M0m_partial input; M0m input; V input
function A_partial = A_partial(q_m,M0,M0_partial,M0m_partial,M0m,V)
% Calculates the C_hat_m matrix from base pose and arm joint angles

n=length(q_m);
b=length(V);

% Find partial of connection A to each joint angle
A_partial=zeros(b,n,n);

temp1=zeros(b,n);
temp2=zeros(b,n);
temp3=zeros(b,n);

for i=1:n
    temp1=M0\(M0_partial(:,:,i));
    temp2=M0\M0m;
    temp3=M0\(M0m_partial(:,:,i));
    A_partial(1:b,1:n,i)=-temp1*temp2+temp3; % Equation 122
end

== matlab function MMMS_v3/Feedback Transformation/Inverse Dynamics1/C_hat/C_hat1 ==
  data: q_m input; Mm_hat_partial input; q_dot_m input; C_hat output
function C_hat = C_hat(q_m, Mm_hat_partial,q_dot_m)
% Calculates the C_hat_m matrix from base pose and arm joint angles

n=length(q_m);


% Calculate C_hat matrix
C_temp1=zeros(n,n);
C_temp2=zeros(n,n);
C_hat=zeros(n,n);
for i=1:n
    C_temp1=C_temp1+squeeze(Mm_hat_partial(1:n,1:n,i)).*q_dot_m(i); % nxn by scalar
    C_temp2(i,1:n)=0.5*transpose(q_dot_m)*squeeze(Mm_hat_partial(1:n,1:n,i)); %1xn by nxn 
end

C_hat=C_temp1-C_temp2;

== matlab function MMMS_v3/Feedback Transformation/Inverse Dynamics1/C_hat/Lm_partials/Lm0partial ==
  data: q_m input; Lm0_partial output; Xi_m input; iota0 input
function Lm0_partial = Lm0_partial(q_m,Xi_m,iota0)
% Calculates the C_hat_m matrix from base pose and arm joint angles

n=length(q_m);

% Find partial of Lm to joint angles
Lm0_partial=zeros(6*n,6,n); % 6nx6xn
for i=1:n
    for j=1:n
        Lm0_partial(6*(j-1)+1:6*j,1:6,i)=Ad_partial(j,1,i,Xi_m,q_m,iota0); % equation 114 of TRO paper
    end
end

%%%%%%%%%%%%%%%%%%%%%%%%%%%%%%%%%%%%%%%%%%%%%%%%%%%%%%%%%%%%% MUST BE
%%%%%%%%%%%%%%%%%%%%%%%%%%%%%%%%%%%%%%%%%%%%%%%%%%%%%%%%%%%%% CHECKED

== matlab function MMMS_v3/Feedback Transformation/Inverse Dynamics1/C_hat/Lm_partials/Lmpartial ==
  data: q_m input; Lm_partial output; Xi_m input; iota0 input
function Lm_partial  = Lm_partial(q_m,Xi_m,iota0)
% Calculates the C_hat_m matrix from base pose and arm joint angles

n=length(q_m);

% Find partial of Lm0 to joint angles
Lm_partial=zeros(6*n,6*n,n); % 6nx6xn
for i=1:n
    Lm_partial(:,:,i)=zeros(6*n,6*n);
    for j=2:n
        for k=2:n
            if j>i && i>=k
                Lm_partial(6*(j-1)+1:6*j,6*(k-2)+1:6*(k-1),i)=Ad_partial(j,k,i,Xi_m,q_m,iota0); % equation 81 of TRO paper
            elseif i==j && i>=k
                Lm_partial(6*(j-1)+1:6*j,6*(k-2)+1:6*(k-1),i)=Ad_partial(j,k,i,Xi_m,q_m,iota0); % equation 81 of TRO paper
            else
                Lm_partial(6*(j-1)+1:6*(j-1)+6,6*(k-2)+1:6*(k-2)+6,i)=zeros(6,6);
            end

        end
    end
end

== matlab function MMMS_v3/MMS2/collect positions ==
  data: p_ni output; p_n2 input; p_n3 input; p_n4 input; p_n5 input; g_n0 input
function p_ni = collect_positions(p_n2,p_n3,p_n4,p_n5, g_n0)

% R_0n=g_n0(1:3,1:3);
% p_0n=g_n0(1:3,4);

% p_joints=zeros(3,5);
p_ni=[p_n2 p_n3 p_n4  p_n5];


% p_joints=p_joints_temp(1:3,:);

== matlab function MMMS_v3/Feedback Transformation/Inverse Dynamics1/C_hat/M_partials/ M0partial ==
  data: q_m input; M0_partial output; Lm0 input; V input; iota0 input; diag_Mm input; Lm0_partial input
function M0_partial = M0_partial(q_m,Lm0,V,iota0,diag_Mm,Lm0_partial)
% Calculates the C_hat_m matrix from base pose and arm joint angles

n=length(q_m);
b=length(V);

% Find partial of M0 to joint angles
M0_partial=zeros(b,b,n); %initiate
for i=1:n
    temp1=transpose(Lm0_partial(1:end,1:end,i))*diag_Mm*Lm0;
    temp2=transpose(Lm0)*diag_Mm*Lm0_partial(1:end,1:end,i);
    M0_partial(1:b,1:b,i)= iota0'*(temp1+temp2)*iota0; %6x6 %equation 117 of TRO
end

== matlab function MMMS_v3/Feedback Transformation/Inverse Dynamics1/C_hat/M_partials/M0mpartial ==
  data: q_m input; M0m_partial output; V input; Lm input; Lm0 input; iota0 input; diag_Mm input; Lm0_partial input; Lm_partial input; Xi_m_matrix input
function M0m_partial = M0m_partial(q_m,V,Lm,Lm0,iota0,diag_Mm,Lm0_partial,Lm_partial, Xi_m_matrix)
% Calculates the C_hat_m matrix from base pose and arm joint angles

n=length(q_m);
b=length(V);

% Find partial of M0m to joint angles
M0m_partial=zeros(b,n,n);
for i=1:n
    temp1=transpose(Lm0_partial(1:end,1:end,i))*diag_Mm*Lm;
    temp2=transpose(Lm0)*diag_Mm*Lm_partial(1:end,1:end,i);
    M0m_partial(1:b,1:n,i)= iota0'*(temp1+temp2)*Xi_m_matrix; % equation 118 of TRO paper
end

== matlab function MMMS_v3/Feedback Transformation/Inverse Dynamics1/C_hat/M_partials/Mmpartial ==
  data: q_m input; Mm_partial output; Xi_m_matrix input; Lm input; diag_Mm input; Lm_partial input
function Mm_partial = Mm_partial(q_m,Xi_m_matrix,Lm,diag_Mm,Lm_partial)
% Calculates the C_hat_m matrix from base pose and arm joint angles

n=length(q_m);

% find the non-generalized arm mass matrix'x derivative to joint angles
Mm_partial=zeros(n,n,n);
for i=1:n
    temp=   transpose(Lm_partial(1:6*n,1:6*n,i))*diag_Mm*Lm  +   transpose(Lm)*diag_Mm*Lm_partial(1:6*n,1:6*n,i);
    Mm_partial(1:n,1:n,i)=transpose(Xi_m_matrix)*temp*Xi_m_matrix; %calcualte the derivative of not-augmented arm mass matrix from equation 120 of TRO paper
end

== matlab function MMMS_v3/Feedback Transformation/Inverse Dynamics1/C_hat/Mm_hat_partial ==
  data: q_m input; AMA_partial input; Mm_hat_partial output; Mm_partial input
function Mm_hat_partial = Mm_hat_partial(q_m, AMA_partial, Mm_partial)
% Calculates the C_hat_m matrix from base pose and arm joint angles

n=length(q_m);

% find the generalized arm mass matrix'x derivative to joint angles
Mm_hat_partial=zeros(n,n,n);
for i=1:n
    Mm_hat_partial(1:n,1:n,i)=Mm_partial(1:n,1:n,i)-AMA_partial(1:n,1:n,i); %calcualte the derivative of augmented arm mass matrix from equation 119 of TRO paper
end

== matlab function MMMS_v3/Feedback Transformation/Inverse Dynamics1/C_hat1/AMA_partial ==
  data: q_m input; AMA_partial output; M0 input; A input; A_partial input; V input; M0_partial input
function AMA_partial = AMA_partial(q_m,M0,A,A_partial,V,M0_partial)
% Calculates the C_hat_m matrix from base pose and arm joint angles

n=length(q_m);
b=length(V);

% find the temp intermediate term
AMA_partial=zeros(n,n,n);
for i=1:n
    AMA_partial(1:n,1:n,i)=transpose(A_partial(1:end,1:end,i))*M0*A+transpose(A)*M0_partial(1:end,1:end,i)*A+transpose(A)*M0*A_partial(1:end,1:end,i); %calcualte the derivative of not-augmented arm mass matrix from equation 121 of TRO paper
end

== matlab function MMMS_v3/Feedback Transformation/Inverse Dynamics1/C_hat1/A_partial ==
  data: q_m input; A_partial output; M0 input; M0_partial input; M0m_partial input; M0m input; V input
function A_partial = A_partial(q_m,M0,M0_partial,M0m_partial,M0m,V)
% Calculates the C_hat_m matrix from base pose and arm joint angles

n=length(q_m);
b=length(V);

% Find partial of connection A to each joint angle
A_partial=zeros(b,n,n);

temp1=zeros(b,n);
temp2=zeros(b,n);
temp3=zeros(b,n);

for i=1:n
    temp1=M0\M0_partial(1:end,1:end,i);
    temp2=M0\M0m;
    temp3=M0\M0m_partial(1:end,1:end,i);
    A_partial(1:b,1:n,i)=-temp1*temp2+temp3; % Equation 122
end

== matlab function MMMS_v3/Feedback Transformation/Inverse Dynamics1/C_hat1/A_partial_par ==
  data: q_m input; A_partial_par output; M0 input; M0_partial input; M0m_partial input; M0m input; V input; M0_partial_par input; M0m_partial_par input
function A_partial_par = A_partial_par(q_m,M0,M0_partial,M0m_partial,M0m,V,M0_partial_par,M0m_partial_par)
% Calculates the C_hat_m matrix from base pose and arm joint angles

n=length(q_m);
b=length(V);

% Find partial of connection A to each joint angle
A_partial_par=zeros(b,n,n,n);

temp1=zeros(b,n);
temp2=zeros(b,n);
temp3=zeros(b,n);

for i=1:n
    for s=1:n
        temp1=M0\M0_partial(1:end,1:end,i);
        temp2=M0\M0_partial(1:end,1:end,s);
        temp3=M0\M0m;
        temp4=M0\M0m_partial(1:end,1:end,i);
        temp5=M0\M0m_partial(1:end,1:end,s);
        A_partial_par(1:b,1:n,i,s)=(M0\     (M0_partial(1:end,1:end,s)*temp1 -M0_partial_par(1:end,1:end,i,s) +M0_partial(1:end,1:end,i)*temp2)           )*temp3 ...
            +M0\(-M0_partial(1:end,1:end,i)*temp5-M0_partial(1:end,1:end,s)*temp4+M0m_partial_par(1:end,1:end,i,s)); % Equation 122????????
    end 
end

== matlab function MMMS_v3/Feedback Transformation/Inverse Dynamics1/C_hat1/C_hat ==
  data: q_m input; Mm_hat_partial input; q_dot_m input; C_hat output
function C_hat = C_hat(q_m, Mm_hat_partial,q_dot_m)
% Calculates the C_hat_m matrix from base pose and arm joint angles

n=length(q_m);


% Calculate C_hat matrix
C_temp1=zeros(n,n);
C_temp2=zeros(n,n);
C_hat=zeros(n,n);
for i=1:n
    C_temp1=C_temp1+squeeze(Mm_hat_partial(1:n,1:n,i)).*q_dot_m(i); % nxn by scalar
    C_temp2(i,1:n)=0.5*transpose(q_dot_m)*squeeze(Mm_hat_partial(1:n,1:n,i)); %1xn by nxn 
end

C_hat=C_temp1-C_temp2;

== matlab function MMMS_v3/Inverse Dynamics/A_dot ==
  data: A_partial input; q_m_dot input; A_dot output
function A_dot = fcn(A_partial, q_m_dot)
n=length(q_m_dot);

A_dot=zeros(6,n);
for i=1:n
    A_dot=A_dot+A_partial(:,:,i).*q_m_dot(i);
end

== matlab function MMMS_v3/Inverse Dynamics/C_hat/AMA_partial ==
  data: q_m input; AMA_partial output; M0 input; A input; A_partial input; V input; M0_partial input
function AMA_partial = AMA_partial(q_m,M0,A,A_partial,V,M0_partial)
% Calculates the C_hat_m matrix from base pose and arm joint angles

n=length(q_m);
b=length(V);

% find the temp intermediate term
AMA_partial=zeros(n,n,n);
for i=1:n
    AMA_partial(1:n,1:n,i)=transpose(A_partial(1:end,1:end,i))*M0*A+transpose(A)*M0_partial(1:end,1:end,i)*A+transpose(A)*M0*A_partial(1:end,1:end,i); %calcualte the derivative of not-augmented arm mass matrix from equation 121 of TRO paper
end

== matlab function MMMS_v3/Controller23/Filter/Triggered Subsystem/MATLAB Function ==
  data: Z input; X_pos_out output double; Dt input; Mass_matrix input; X_pos input; mu_vector input; P_pos input; Q input; R input; P_pos_out output double
function [X_pos_out,P_pos_out] = fcn(Z,Dt,Mass_matrix,X_pos,mu_vector,P_pos,Q,R)
% X_pos_out=eye(4);
% P_pos_out=zeros(6);
mu_vector = [mu_vector(4:6);mu_vector(1:3)];

Omega = Dt*inv(Mass_matrix)*Adjoint_EKF(inv(X_pos))*mu_vector;
D   = DMatrix(X_pos,Dt,Mass_matrix,mu_vector);
F   = Adjoint_EKF(expm(wedge_EKF(-Omega)))...
                   +Right_Jacob_SE(Omega)*D; 
X_pri = X_pos*expm(wedge_EKF(Omega));
P_pri = F*P_pos*F'...
                   +Right_Jacob_SE(Omega)*Q*Right_Jacob_SE(Omega)';
nu        = LieAlgebra(inv(h_fcn(X_pri))*Z);
H = [1 0 0 0 0 0; 0 1 0 0 0 0; 0 0 1 0 0 0; 0 0 0 1 0 0;0 0 0 0 1 0;0 0 0 0 0 1];
K     = P_pri*H'*inv(H*P_pri*H'+R);
X_pos_out = X_pri*real(expm(wedge_EKF( K*nu))) ;
P_pos_out = real(Right_Jacob_SE(K*nu)*(eye(6)-K*H)...
                   *P_pri*Right_Jacob_SE(K*nu)');

== matlab function MMMS_v3/Inverse Dynamics/C_hat/A_partial ==
  data: q_m input; A_partial output; M0 input; M0_partial input; M0m_partial input; M0m input; V input
function A_partial = A_partial(q_m,M0,M0_partial,M0m_partial,M0m,V)
% Calculates the C_hat_m matrix from base pose and arm joint angles

n=length(q_m);
b=length(V);

% Find partial of connection A to each joint angle
A_partial=zeros(b,n,n);

temp1=zeros(b,n);
temp2=zeros(b,n);
temp3=zeros(b,n);

for i=1:n
    temp1=M0\(M0_partial(:,:,i));
    temp2=M0\M0m;
    temp3=M0\(M0m_partial(:,:,i));
    A_partial(1:b,1:n,i)=-temp1*temp2+temp3; % Equation 122
end

== matlab function MMMS_v3/Inverse Dynamics/C_hat/C_hat1 ==
  data: q_m input; Mm_hat_partial input; q_dot_m input; C_hat output
function C_hat = C_hat(q_m, Mm_hat_partial,q_dot_m)
% Calculates the C_hat_m matrix from base pose and arm joint angles

n=length(q_m);


% Calculate C_hat matrix
C_temp1=zeros(n,n);
C_temp2=zeros(n,n);
C_hat=zeros(n,n);
for i=1:n
    C_temp1=C_temp1+squeeze(Mm_hat_partial(1:n,1:n,i)).*q_dot_m(i); % nxn by scalar
    C_temp2(i,1:n)=0.5*transpose(q_dot_m)*squeeze(Mm_hat_partial(1:n,1:n,i)); %1xn by nxn 
end

C_hat=C_temp1-C_temp2;
